simulink model "SF009A_DutyCycThermProtn"  (R2013b)
settings: Solver=FixedStepDiscrete  SolverMode=SingleTasking  StartTime=0.0  StopTime=1  FixedStep=0.1  RelTol=1e-3
undefined symbols (not defined in the file): AbsltTThermLimCnt, ARCHGLBPRM_100MILLISEC_SEC_F32, CTRLRANDCUTFLT_CNT_U08, CTRLRTFLT_CNT_U08, CUTFLT_CNT_U08, DITHERMLIM_MOTNWTMTR_F32, DutyCycExcddCnt, DutyCycThermProtnAbsltCtrlTTblX, DutyCycThermProtnAbsltCtrlTTqTblY, DutyCycThermProtnAbsltCuTTblX, DutyCycThermProtnAbsltCuTTqTblY, DutyCycThermProtnAbsltMotVelBreakPt, DutyCycThermProtnAbsltTTqSlewHiLim, DutyCycThermProtnAbsltTTqSlewLoLim, DutyCycThermProtnCtrlT, DutyCycThermProtnCtrlTSeln, DutyCycThermProtnDutyCycFildThd, DutyCycThermProtnIgnOffCtrlEna, DutyCycThermProtnIgnOffMsgWaitTi, DutyCycThermProtnLstTblValNonStall, DutyCycThermProtnLstTblValStall, DutyCycThermProtnMotPrTSeln, DutyCycThermProtnMplr1NonStallTblY, DutyCycThermProtnMplr1StallTblY, DutyCycThermProtnMplr2NonStallTblY, DutyCycThermProtnMplr2StallTblY, DutyCycThermProtnMplr3NonStallTblY, DutyCycThermProtnMplr3StallTblY, DutyCycThermProtnMplr4NonStallTblY, DutyCycThermProtnMplr4StallTblY, DutyCycThermProtnMplr5NonStallTblY, DutyCycThermProtnMplr5StallTblY, DutyCycThermProtnMplr6NonStallTblY, DutyCycThermProtnMplr6StallTblY, DutyCycThermProtnMplrTblX, DutyCycThermProtnMplrTSeln, DutyCycThermProtnSlowFilTSeln, DutyCycThermProtnThermLoadLimTblX, DutyCycThermProtnThermLoadLimTblY, DutyCycThermProtnTqCmdSlewDwn, DutyCycThermProtnTqCmdSlewUp, FILVALMIN_ULS_F32, IGNTIOFFTHD_CNT_F32, NODEBSTEP_CNT_U16, NtcSts1, NvmGetErrSts1, ONEPERC_ULS_F32, TAU3_SEC_F32, TAU4_SEC_F32, TAU5_SEC_F32, TAU6_SEC_F32, THERMLOADLIMTBLIDX_ULS_U08
libraries: FixdToFloat x13, Fil x12, simulink x11, NxtrLim x10, NxtrMath x8, FloatToFixd x6, NxtrMax x6, NxtrMin x4, NxtrAbslt x2, NxtrNvM x1
(part 6 of 6)

== system SF009A_DutyCycThermProtn/DutyCycThermProtn/DutyCycThermProtnPer1/TempratureLimiting/SetNtc/SetNtcSts ==
  note: Note:
      |
      | - "ISO Fault Debounce Design" Simulink block intent to use here for Simulation purpose only. Do not Code this block
  NtcNr : Inport
  NtcStInfo : Inport  Port=2
  NtcSts : Inport  Port=3
  DebStep : Inport  Port=4
  Copyright1 : Subsystem  Description=|  RequirementInfo={} %GIDa_eb45801b_6e45_4d0e_85d0_27f2c30c63b6  mask(Copyright Information){none=on}
      | Copyright info block.                                               
      |                                                                     
      | Place copyright information at the top of every subsystem in design.
      mask prompts: none "No parameters"
      mask help: Place copyright information at the top of every subsystem in design.
      mask Display:
      | NxtrConf = 'Nexteer Confidential';
      | 
      | sys = bdroot; %handle for the current model ("system")
      | first = get_param(sys,'Created');
      | if(isempty(first))
      |     first = datestr(now,'yyyy');
      | else
      |     first = first(end-3:end);  %year is last four digits
      | end
      | 
      | last = get_param(sys,'LastModifiedDate');
      | if isempty(last)
      |     last = datestr(now,'yyyy');
      | else
      |     last = last(end-3:end);
      | end
      | 
      | if strcmp(first,last)
      |     fprintf('%s\nCopyright  %s Nexteer',NxtrConf,first);
      | else
      |     fprintf('%s\n%s%s-%s Nexteer',NxtrConf,char(169),first,last);
      | end
  Data Store Write : DataStoreWrite  DataStoreName=AbsltTThermLimCntQlfr
  Data Store Write2 : DataStoreWrite  DataStoreName=AbsltTThermLimCntStInfo
  Data Store Write3 : DataStoreWrite  DataStoreName=AbsltTThermLimCntStsVal
  Data Type Conversion : DataTypeConversion  OutDataTypeStr=Enum: SigQlfr1
  Ground : Ground
  ISO Fault Debounce Design : Stateflow chart  TreatAsAtomicUnit=on
      settings: AttributesFormatString=|
      | Simulation Purpose Only.
      | Do Not Code this block
      | Diagnostic Manager Owns this requirement
  Terminator : Terminator
  Terminator1 : Terminator
  wires:
  NtcNr/1 -> Terminator/1
  NtcStInfo/1 -> Data Store Write2/1, Terminator1/1
  DebStep/1 -> ISO Fault Debounce Design/2(DebStep)
  Ground/1 -> ISO Fault Debounce Design/3(SvcClr)
  NtcSts/1 -> Data Store Write3/1, ISO Fault Debounce Design/1(NtcSts)
  ISO Fault Debounce Design/1(Qualifier) -> Data Type Conversion/1
  Data Type Conversion/1 -> Data Store Write/1

== system SF009A_DutyCycThermProtn/DutyCycThermProtn/DutyCycThermProtnPer1/TempratureLimiting/SetPassdNtc/CopyRight2 ==

== system SF009A_DutyCycThermProtn/DutyCycThermProtn/DutyCycThermProtnPer1/ThermalLimitStatus/DutyCycThermProtnDisabled/CopyRight2 ==

== system SF009A_DutyCycThermProtn/DutyCycThermProtn/DutyCycThermProtnPer1/ThermalLimitStatus/DutyCycThermProtnEnabled /CopyRight2 ==

== system SF009A_DutyCycThermProtn/DutyCycThermProtn/DutyCycThermProtnPer1/ThermalLimitStatus/MaxoutLimiting/CopyRight2 ==

== system SF009A_DutyCycThermProtn/DutyCycThermProtn/DutyCycThermProtnPer1/ThermalLimitStatus/MaxoutLimiting/SetNtcFail ==
  NtcNr : Inport
  NtcStInfo : Inport  Port=2
  NtcSts : Inport  Port=3
  DebStep : Inport  Port=4
  Action Port : ActionPort  ActionType=else
  Copyright1 : Subsystem  Description=|  RequirementInfo={} %GIDa_8d6137ac_426a_4835_9288_59de8ac60212  mask(Copyright Information){none=on}
      | Copyright info block.                                               
      |                                                                     
      | Place copyright information at the top of every subsystem in design.
      mask prompts: none "No parameters"
      mask help: Place copyright information at the top of every subsystem in design.
      mask Display:
      | NxtrConf = 'Nexteer Confidential';
      | 
      | sys = bdroot; %handle for the current model ("system")
      | first = get_param(sys,'Created');
      | if(isempty(first))
      |     first = datestr(now,'yyyy');
      | else
      |     first = first(end-3:end);  %year is last four digits
      | end
      | 
      | last = get_param(sys,'LastModifiedDate');
      | if isempty(last)
      |     last = datestr(now,'yyyy');
      | else
      |     last = last(end-3:end);
      | end
      | 
      | if strcmp(first,last)
      |     fprintf('%s\nCopyright  %s Nexteer',NxtrConf,first);
      | else
      |     fprintf('%s\n%s%s-%s Nexteer',NxtrConf,char(169),first,last);
      | end
  SetNtcSts : Subsystem  RequirementInfo={} %GIDa_fdfb0ccc_741b_4ffc_97ed_944bcf90493a
  wires:
  DebStep/1 -> SetNtcSts/4(DebStep)
  NtcSts/1 -> SetNtcSts/3(NtcSts)
  NtcStInfo/1 -> SetNtcSts/2(NtcStInfo)
  NtcNr/1 -> SetNtcSts/1(NtcNr)

== system SF009A_DutyCycThermProtn/DutyCycThermProtn/DutyCycThermProtnPer1/ThermalLimitStatus/MaxoutLimiting/SetNtcPass ==
  NtcNr : Inport
  NtcStInfo : Inport  Port=2
  NtcSts : Inport  Port=3
  DebStep : Inport  Port=4
  Action Port : ActionPort  ActionType=then
  Copyright1 : Subsystem  Description=|  RequirementInfo={} %GIDa_805612c1_a02e_4620_a20f_eb93e5c11a84  mask(Copyright Information){none=on}
      | Copyright info block.                                               
      |                                                                     
      | Place copyright information at the top of every subsystem in design.
      mask prompts: none "No parameters"
      mask help: Place copyright information at the top of every subsystem in design.
      mask Display:
      | NxtrConf = 'Nexteer Confidential';
      | 
      | sys = bdroot; %handle for the current model ("system")
      | first = get_param(sys,'Created');
      | if(isempty(first))
      |     first = datestr(now,'yyyy');
      | else
      |     first = first(end-3:end);  %year is last four digits
      | end
      | 
      | last = get_param(sys,'LastModifiedDate');
      | if isempty(last)
      |     last = datestr(now,'yyyy');
      | else
      |     last = last(end-3:end);
      | end
      | 
      | if strcmp(first,last)
      |     fprintf('%s\nCopyright  %s Nexteer',NxtrConf,first);
      | else
      |     fprintf('%s\n%s%s-%s Nexteer',NxtrConf,char(169),first,last);
      | end
  SetNtcSts : Subsystem  RequirementInfo={} %GIDa_e6aea97a_d4f1_4b4b_ab02_7f79c2ea91b3
  wires:
  NtcNr/1 -> SetNtcSts/1(NtcNr)
  NtcStInfo/1 -> SetNtcSts/2(NtcStInfo)
  NtcSts/1 -> SetNtcSts/3(NtcSts)
  DebStep/1 -> SetNtcSts/4(DebStep)

== system SF009A_DutyCycThermProtn/DutyCycThermProtn/DutyCycThermProtnPer1/ThermalLimitStatus/ThermLim_DutyCycThermProtnDisabled/CopyRight2 ==

== system SF009A_DutyCycThermProtn/DutyCycThermProtn/DutyCycThermProtnPer1/ThermalLimitStatus/ThermLim_DutyCycThermProtnEnabled/CopyRight2 ==

== system SF009A_DutyCycThermProtn/DutyCycThermProtn/DutyCycThermProtnInit1/PowerOnTasks/InputIgnOffTime/Filt3ExpDecay/CopyRight2 ==

== system SF009A_DutyCycThermProtn/DutyCycThermProtn/DutyCycThermProtnInit1/PowerOnTasks/InputIgnOffTime/Filt4ExpDecay/CopyRight2 ==

== system SF009A_DutyCycThermProtn/DutyCycThermProtn/DutyCycThermProtnInit1/PowerOnTasks/InputIgnOffTime/Filt5ExpDecay/CopyRight2 ==

== system SF009A_DutyCycThermProtn/DutyCycThermProtn/DutyCycThermProtnInit1/PowerOnTasks/InputIgnOffTime/Filt6ExpDecay/CopyRight2 ==

== system SF009A_DutyCycThermProtn/DutyCycThermProtn/DutyCycThermProtnPer1/FiltSVReinit/VehTiVldEnabled/Filt3ExpDecay/CopyRight2 ==

== system SF009A_DutyCycThermProtn/DutyCycThermProtn/DutyCycThermProtnPer1/FiltSVReinit/VehTiVldEnabled/Filt4ExpDecay/CopyRight2 ==

== system SF009A_DutyCycThermProtn/DutyCycThermProtn/DutyCycThermProtnPer1/FiltSVReinit/VehTiVldEnabled/Filt5ExpDecay/CopyRight2 ==

== system SF009A_DutyCycThermProtn/DutyCycThermProtn/DutyCycThermProtnPer1/FiltSVReinit/VehTiVldEnabled/Filt6ExpDecay/CopyRight2 ==

== system SF009A_DutyCycThermProtn/DutyCycThermProtn/DutyCycThermProtnPer1/LoadLimiting/FilterPercMax/DutyCycLevel_DutyCycThermProtnDisabled/CopyRight2 ==

== system SF009A_DutyCycThermProtn/DutyCycThermProtn/DutyCycThermProtnPer1/LoadLimiting/FilterPercMax/DutyCycLevel_DutyCycThermProtnEnabled/CopyRight2 ==

== system SF009A_DutyCycThermProtn/DutyCycThermProtn/DutyCycThermProtnPer1/LoadLimiting/Multiplier/NonStallCondition/CopyRight2 ==

== system SF009A_DutyCycThermProtn/DutyCycThermProtn/DutyCycThermProtnPer1/LoadLimiting/Multiplier/SlowFilTSeln_Mult12Temp/CopyRight2 ==

== system SF009A_DutyCycThermProtn/DutyCycThermProtn/DutyCycThermProtnPer1/LoadLimiting/Multiplier/SlowFilTSeln_Mult36Temp/CopyRight2 ==

== system SF009A_DutyCycThermProtn/DutyCycThermProtn/DutyCycThermProtnPer1/LoadLimiting/Multiplier/StallCondition/CopyRight2 ==

== system SF009A_DutyCycThermProtn/DutyCycThermProtn/DutyCycThermProtnPer1/LoadLimiting/ThermalLoadLimit/DutyCycleLevel_LstTblValNonStall/CopyRight2 ==

== system SF009A_DutyCycThermProtn/DutyCycThermProtn/DutyCycThermProtnPer1/LoadLimiting/ThermalLoadLimit/DutyCycleLevel_LstTblValStall/CopyRight2 ==

== system SF009A_DutyCycThermProtn/DutyCycThermProtn/DutyCycThermProtnPer1/TemperatureSelection/Mult12T_DiagcStsLimdTPrfmncDisabled/CtrlTSelnDisabled/CopyRight2 ==

== system SF009A_DutyCycThermProtn/DutyCycThermProtn/DutyCycThermProtnPer1/TemperatureSelection/Mult12T_DiagcStsLimdTPrfmncDisabled/CtrlTSelnEnabled/CopyRight2 ==

== system SF009A_DutyCycThermProtn/DutyCycThermProtn/DutyCycThermProtnPer1/TemperatureSelection/Mult36T_DiagcStsLimdTPrfmncDisabled/MotPrTSelnDisabled/CopyRight2 ==

== system SF009A_DutyCycThermProtn/DutyCycThermProtn/DutyCycThermProtnPer1/TemperatureSelection/Mult36T_DiagcStsLimdTPrfmncDisabled/MotPrTSelnEnabled/CopyRight2 ==

== system SF009A_DutyCycThermProtn/DutyCycThermProtn/DutyCycThermProtnPer1/TempratureLimiting/SetNtc/SetNtcSts/Copyright1 ==

== system SF009A_DutyCycThermProtn/DutyCycThermProtn/DutyCycThermProtnPer1/ThermalLimitStatus/MaxoutLimiting/SetNtcFail/Copyright1 ==

== system SF009A_DutyCycThermProtn/DutyCycThermProtn/DutyCycThermProtnPer1/ThermalLimitStatus/MaxoutLimiting/SetNtcFail/SetNtcSts ==
  note: Note:
      |
      | - "ISO Fault Debounce Design" Simulink block intent to use here for Simulation purpose only. Do not Code this block
  NtcNr : Inport
  NtcStInfo : Inport  Port=2
  NtcSts : Inport  Port=3
  DebStep : Inport  Port=4
  Copyright1 : Subsystem  Description=|  RequirementInfo={} %GIDa_c559b048_8a37_4c40_bbc3_34832b025652  mask(Copyright Information){none=on}
      | Copyright info block.                                               
      |                                                                     
      | Place copyright information at the top of every subsystem in design.
      mask prompts: none "No parameters"
      mask help: Place copyright information at the top of every subsystem in design.
      mask Display:
      | NxtrConf = 'Nexteer Confidential';
      | 
      | sys = bdroot; %handle for the current model ("system")
      | first = get_param(sys,'Created');
      | if(isempty(first))
      |     first = datestr(now,'yyyy');
      | else
      |     first = first(end-3:end);  %year is last four digits
      | end
      | 
      | last = get_param(sys,'LastModifiedDate');
      | if isempty(last)
      |     last = datestr(now,'yyyy');
      | else
      |     last = last(end-3:end);
      | end
      | 
      | if strcmp(first,last)
      |     fprintf('%s\nCopyright  %s Nexteer',NxtrConf,first);
      | else
      |     fprintf('%s\n%s%s-%s Nexteer',NxtrConf,char(169),first,last);
      | end
  Data Store Write : DataStoreWrite  DataStoreName=DutyCycExcddCntQlfr
  Data Store Write2 : DataStoreWrite  DataStoreName=DutyCycExcddCntStInfo
  Data Store Write3 : DataStoreWrite  DataStoreName=DutyCycExcddCntStsVal
  Data Type Conversion : DataTypeConversion  OutDataTypeStr=Enum: SigQlfr1
  Ground : Ground
  ISO Fault Debounce Design : Stateflow chart  TreatAsAtomicUnit=on
      settings: AttributesFormatString=|
      | Simulation Purpose Only.
      | Do Not Code this block
      | Diagnostic Manager Owns this requirement
  Terminator : Terminator
  Terminator1 : Terminator
  wires:
  Data Type Conversion/1 -> Data Store Write/1
  ISO Fault Debounce Design/1(Qualifier) -> Data Type Conversion/1
  NtcSts/1 -> Data Store Write3/1, ISO Fault Debounce Design/1(NtcSts)
  Ground/1 -> ISO Fault Debounce Design/3(SvcClr)
  DebStep/1 -> ISO Fault Debounce Design/2(DebStep)
  NtcStInfo/1 -> Terminator1/1, Data Store Write2/1
  NtcNr/1 -> Terminator/1

== system SF009A_DutyCycThermProtn/DutyCycThermProtn/DutyCycThermProtnPer1/ThermalLimitStatus/MaxoutLimiting/SetNtcPass/Copyright1 ==

== system SF009A_DutyCycThermProtn/DutyCycThermProtn/DutyCycThermProtnPer1/ThermalLimitStatus/MaxoutLimiting/SetNtcPass/SetNtcSts ==
  note: Note:
      |
      | - "ISO Fault Debounce Design" Simulink block intent to use here for Simulation purpose only. Do not Code this block
  NtcNr : Inport
  NtcStInfo : Inport  Port=2
  NtcSts : Inport  Port=3
  DebStep : Inport  Port=4
  Copyright1 : Subsystem  Description=|  RequirementInfo={} %GIDa_51294eaf_cd8b_4a83_995e_49de41be9351  mask(Copyright Information){none=on}
      | Copyright info block.                                               
      |                                                                     
      | Place copyright information at the top of every subsystem in design.
      mask prompts: none "No parameters"
      mask help: Place copyright information at the top of every subsystem in design.
      mask Display:
      | NxtrConf = 'Nexteer Confidential';
      | 
      | sys = bdroot; %handle for the current model ("system")
      | first = get_param(sys,'Created');
      | if(isempty(first))
      |     first = datestr(now,'yyyy');
      | else
      |     first = first(end-3:end);  %year is last four digits
      | end
      | 
      | last = get_param(sys,'LastModifiedDate');
      | if isempty(last)
      |     last = datestr(now,'yyyy');
      | else
      |     last = last(end-3:end);
      | end
      | 
      | if strcmp(first,last)
      |     fprintf('%s\nCopyright  %s Nexteer',NxtrConf,first);
      | else
      |     fprintf('%s\n%s%s-%s Nexteer',NxtrConf,char(169),first,last);
      | end
  Data Store Write : DataStoreWrite  DataStoreName=DutyCycExcddCntQlfr
  Data Store Write2 : DataStoreWrite  DataStoreName=DutyCycExcddCntStInfo
  Data Store Write3 : DataStoreWrite  DataStoreName=DutyCycExcddCntStsVal
  Data Type Conversion : DataTypeConversion  OutDataTypeStr=Enum: SigQlfr1
  Ground : Ground
  ISO Fault Debounce Design : Stateflow chart  TreatAsAtomicUnit=on
      settings: AttributesFormatString=|
      | Simulation Purpose Only.
      | Do Not Code this block
      | Diagnostic Manager Owns this requirement
  Terminator : Terminator
  Terminator1 : Terminator
  wires:
  Data Type Conversion/1 -> Data Store Write/1
  ISO Fault Debounce Design/1(Qualifier) -> Data Type Conversion/1
  NtcSts/1 -> Data Store Write3/1, ISO Fault Debounce Design/1(NtcSts)
  Ground/1 -> ISO Fault Debounce Design/3(SvcClr)
  DebStep/1 -> ISO Fault Debounce Design/2(DebStep)
  NtcStInfo/1 -> Terminator1/1, Data Store Write2/1
  NtcNr/1 -> Terminator/1

== system SF009A_DutyCycThermProtn/DutyCycThermProtn/DutyCycThermProtnPer1/ThermalLimitStatus/MaxoutLimiting/SetNtcFail/SetNtcSts/Copyright1 ==

== system SF009A_DutyCycThermProtn/DutyCycThermProtn/DutyCycThermProtnPer1/ThermalLimitStatus/MaxoutLimiting/SetNtcPass/SetNtcSts/Copyright1 ==

== stateflow chart SF009A_DutyCycThermProtn/DutyCycThermProtn/DutyCycThermProtnPer1/TempratureLimiting/SetNtc/SetNtcSts/ISO Fault Debounce Design ==
  note: NTCSTS_PASSD           (0)
      | NTCSTS_FAILD             (1)
      | NTCSTS_PREPASSD   (2)
      | NTCSTS_PREFAILD     (3)
      |
      | SIGQLFR_NORES        (0)
      | SIGQLFR_PASSD         (1)
      | SIGQLFR_FAILD           (2)
  note: Pass Loop
  note: Fail Loop
  note: 
  (default) -> (junction 89)
  (junction 89) -> (junction 95) [order 1] : [NtcSts ==3]
  (junction 89) -> (junction 93) [order 2] : [NtcSts ==2]
  (junction 89) -> (junction 141) [order 3] : [NtcSts ==1]
      | { ErrAcc = 200;
      | Qualifier =2;
      |  }
  (junction 89) -> (junction 141) [order 4] : [NtcSts ==0]
      | { ErrAcc = 0;
      | Qualifier=1;
      | }
  (junction 95) -> (junction 103) [order 2]
  (junction 95) -> (junction 111) [order 1] : [ErrAcc <=0]
      | {ErrAcc = DebStep;}
  (junction 93) -> (junction 123) [order 2] : {
      | ErrAcc = ErrAcc - DebStep;
      | }
  (junction 93) -> (junction 123) [order 1] : [(ErrAcc - DebStep) <= 0]
      | { ErrAcc = 0;
      | Qualifier=1;
      | }
  (junction 103) -> (junction 111) [order 1] : [(ErrAcc + DebStep) <200]
      | {ErrAcc = ErrAcc + DebStep;}
  (junction 103) -> (junction 111) [order 2] : {ErrAcc = 200;
      | Qualifier =2;}
  (junction 123) -> (junction 141)
  (junction 111) -> (junction 141)
  (junction 141) -> (junction 159) [order 2]
  (junction 141) -> (junction 159) [order 1] : [SvcClr ==0]
  data: NtcSts input Enum: NtcSts1; Qualifier output uint8; DebStep input; ErrAcc local single; SvcClr input

== stateflow chart SF009A_DutyCycThermProtn/DutyCycThermProtn/DutyCycThermProtnPer1/ThermalLimitStatus/MaxoutLimiting/SetNtcFail/SetNtcSts/ISO Fault Debounce Design ==
  note: NTCSTS_PASSD           (0)
      | NTCSTS_FAILD             (1)
      | NTCSTS_PREPASSD   (2)
      | NTCSTS_PREFAILD     (3)
      |
      | SIGQLFR_NORES        (0)
      | SIGQLFR_PASSD         (1)
      | SIGQLFR_FAILD           (2)
  note: Pass Loop
  note: Fail Loop
  note: 
  (default) -> (junction 89)
  (junction 89) -> (junction 95) [order 1] : [NtcSts ==3]
  (junction 89) -> (junction 93) [order 2] : [NtcSts ==2]
  (junction 89) -> (junction 141) [order 3] : [NtcSts ==1]
      | { ErrAcc = 200;
      | Qualifier =2;
      |  }
  (junction 89) -> (junction 141) [order 4] : [NtcSts ==0]
      | { ErrAcc = 0;
      | Qualifier=1;
      | }
  (junction 95) -> (junction 103) [order 2]
  (junction 95) -> (junction 111) [order 1] : [ErrAcc <=0]
      | {ErrAcc = DebStep;}
  (junction 93) -> (junction 123) [order 2] : {
      | ErrAcc = ErrAcc - DebStep;
      | }
  (junction 93) -> (junction 123) [order 1] : [(ErrAcc - DebStep) <= 0]
      | { ErrAcc = 0;
      | Qualifier=1;
      | }
  (junction 103) -> (junction 111) [order 1] : [(ErrAcc + DebStep) <200]
      | {ErrAcc = ErrAcc + DebStep;}
  (junction 103) -> (junction 111) [order 2] : {ErrAcc = 200;
      | Qualifier =2;}
  (junction 123) -> (junction 141)
  (junction 111) -> (junction 141)
  (junction 141) -> (junction 159) [order 2]
  (junction 141) -> (junction 159) [order 1] : [SvcClr ==0]
  data: NtcSts input Enum: NtcSts1; Qualifier output uint8; DebStep input; ErrAcc local single; SvcClr input

== stateflow chart SF009A_DutyCycThermProtn/DutyCycThermProtn/DutyCycThermProtnPer1/ThermalLimitStatus/MaxoutLimiting/SetNtcPass/SetNtcSts/ISO Fault Debounce Design ==
  note: NTCSTS_PASSD           (0)
      | NTCSTS_FAILD             (1)
      | NTCSTS_PREPASSD   (2)
      | NTCSTS_PREFAILD     (3)
      |
      | SIGQLFR_NORES        (0)
      | SIGQLFR_PASSD         (1)
      | SIGQLFR_FAILD           (2)
  note: Pass Loop
  note: Fail Loop
  note: 
  (default) -> (junction 89)
  (junction 89) -> (junction 95) [order 1] : [NtcSts ==3]
  (junction 89) -> (junction 93) [order 2] : [NtcSts ==2]
  (junction 89) -> (junction 141) [order 3] : [NtcSts ==1]
      | { ErrAcc = 200;
      | Qualifier =2;
      |  }
  (junction 89) -> (junction 141) [order 4] : [NtcSts ==0]
      | { ErrAcc = 0;
      | Qualifier=1;
      | }
  (junction 95) -> (junction 103) [order 2]
  (junction 95) -> (junction 111) [order 1] : [ErrAcc <=0]
      | {ErrAcc = DebStep;}
  (junction 93) -> (junction 123) [order 2] : {
      | ErrAcc = ErrAcc - DebStep;
      | }
  (junction 93) -> (junction 123) [order 1] : [(ErrAcc - DebStep) <= 0]
      | { ErrAcc = 0;
      | Qualifier=1;
      | }
  (junction 103) -> (junction 111) [order 1] : [(ErrAcc + DebStep) <200]
      | {ErrAcc = ErrAcc + DebStep;}
  (junction 103) -> (junction 111) [order 2] : {ErrAcc = 200;
      | Qualifier =2;}
  (junction 123) -> (junction 141)
  (junction 111) -> (junction 141)
  (junction 141) -> (junction 159) [order 2]
  (junction 141) -> (junction 159) [order 1] : [SvcClr ==0]
  data: NtcSts input Enum: NtcSts1; Qualifier output uint8; DebStep input; ErrAcc local single; SvcClr input
